simulink model "SL_Bsp_01"  (R2020a)
settings: Solver=VariableStepAuto  StartTime=0.0  StopTime=10.0  RelTol=1e-3
values from neighbouring files (symbols this model uses):
  A = [-Rs/Ls,    0,      0,        0 ... (first row only)    [bldc_motor.m]    (also in test_simulink.m = 0.323; test_simulink_0.m = 2; ueb_simulink_ofen.m = 0.323)
  I1_0 = -A    (= -2)    [test_simulink_0.m]
settings Model: Creator=Horst  LastModifiedBy=Horst
settings DataIOCC: ReturnWorkspaceOutputs=off

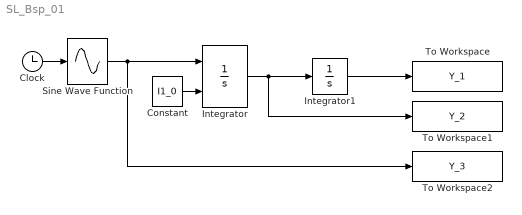
== system SL_Bsp_01 ==
  Clock : Clock
  Constant : Constant  Value=I1_0
  Integrator : Integrator  InitialConditionSource=external  InitialCondition=-1
  Integrator1 : Integrator
  Sine Wave Function : Sin  TimeSource=Use external signal  Amplitude=A  SampleTime=0
  To Workspace : ToWorkspace  VariableName=Y_1  SampleTime=-1
  To Workspace1 : ToWorkspace  VariableName=Y_2  SampleTime=-1
  To Workspace2 : ToWorkspace  VariableName=Y_3  SampleTime=-1
  wires:
  Sine Wave Function/1 -> To Workspace2/1, Integrator/1
  Integrator/1 -> To Workspace1/1, Integrator1/1
  Integrator1/1 -> To Workspace/1
  Clock/1 -> Sine Wave Function/1
  Constant/1 -> Integrator/2
